simulink model "Sway_control_test"  (R2021a)
settings: Solver=VariableStepAuto  StartTime=0.0  StopTime=100.0  MaxStep=1e-3  RelTol=1e-3
values from neighbouring files (symbols this model uses):
  bEtd = (btd + btm*it^2)/rtd^2    (= 21607.2)    [Data.m]
  g = 9.80665    [Data.m]
  it = 30    [Data.m]
  MEtd = (Jtd + Jtm_tb*it^2)/rtd^2    (= 30000)    [Data.m]
  Ms = 15000    [Data.m]
  rtd = 0.5    [Data.m]
settings Model: Creator=ThnkPad  LastModifiedBy=ThnkPad

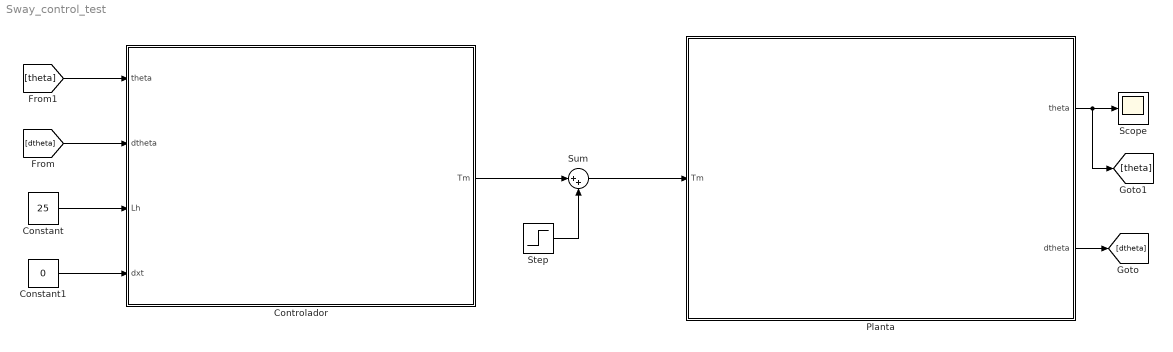
== system Sway_control_test ==
  Constant : Constant  Value=25
  Constant1 : Constant  Value=0
  Controlador : Subsystem
  Planta : Subsystem
  Scope : Scope
  Step : Step  Before=100  After=0  SampleTime=0
  Sum : Sum  Inputs=|++
  wires:
  Planta/1(theta) -> [theta], Scope/1
  Sum/1 -> Planta/1(Tm)
  Controlador/1(Tm) -> Sum/1
  Step/1 -> Sum/2
  Constant/1 -> Controlador/3(Lh)
  Planta/2(dtheta) -> [dtheta]
  [dtheta] -> Controlador/2(dtheta)
  [theta] -> Controlador/1(theta)
  Constant1/1 -> Controlador/4(dxt)

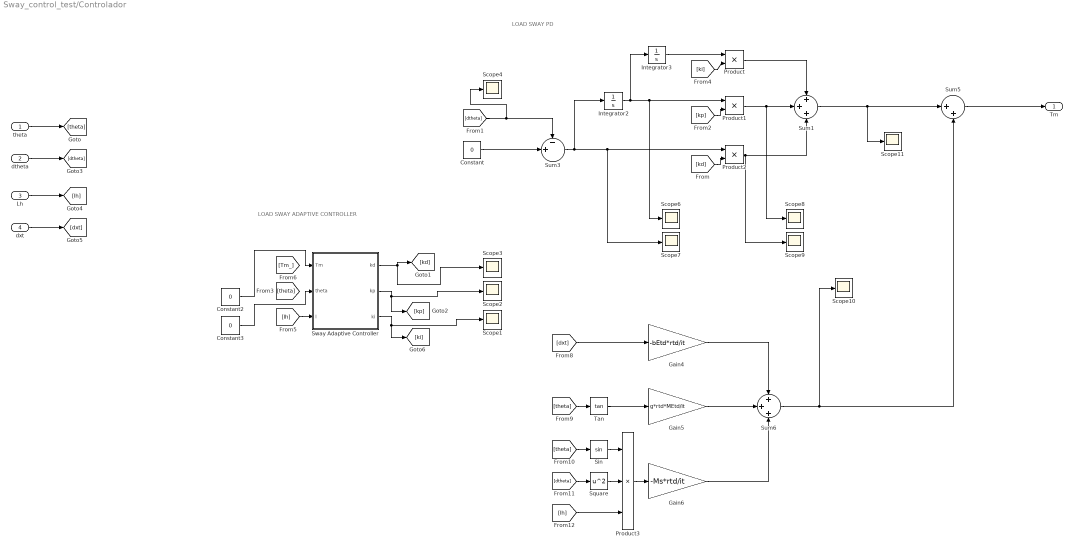
== system Sway_control_test/Controlador ==
  note: LOAD SWAY ADAPTIVE CONTROLLER
  note: LOAD SWAY PD
  theta : Inport
  dtheta : Inport  Port=2
  Lh : Inport  Port=3
  dxt : Inport  Port=4
  Constant : Constant  Value=0
  Constant2 : Constant  Value=0
  Constant3 : Constant  Value=0
  Gain4 : Gain  Gain=-bEtd*rtd/it
  Gain5 : Gain  Gain=g*rtd*MEtd/it
  Gain6 : Gain  Gain=-Ms*rtd/it
  Integrator2 : Integrator
  Integrator3 : Integrator
  Product : Product
  Product1 : Product
  Product2 : Product
  Product3 : Product  Inputs=3
  Scope{1..4,6..11} (10 alike) : Scope
  Sin : Trigonometry
  Square : Math  Operator=square  SaturateOnIntegerOverflow=on
  Sum1 : Sum  Inputs=+++
  Sum3 : Sum  Inputs=-+|
  Sum5 : Sum  Inputs=|++
  Sum6 : Sum  Inputs=+++
  Sway Adaptive Controller : Subsystem
  Tan : Trigonometry  Operator=tan
  Tm : Outport
  wires:
  Sway Adaptive Controller/3(ki) -> Scope1/1, [ki]
  Sway Adaptive Controller/2(kp) -> [kp], Scope2/1
  Integrator2/1 -> Integrator3/1, Scope6/1, Product1/1
  [dxt] -> Gain4/1
  [theta] -> Sin/1
  Product1/1 -> Scope8/1, Sum1/2
  Sum6/1 -> Sum5/2, Scope10/1
  Integrator3/1 -> Product/1
  [kp] -> Product1/2
  [dtheta] -> Scope4/1, Sum3/1
  Sway Adaptive Controller/1(kd) -> Scope3/1, [kd]
  Sum3/1 -> Scope7/1, Product2/1, Integrator2/1
  [lh] -> Sway Adaptive Controller/3(l)
  Sin/1 -> Product3/1
  Product3/1 -> Gain6/1
  Product2/1 -> Sum1/3, Scope9/1
  Sum5/1 -> Tm/1
  Constant2/1 -> Sway Adaptive Controller/1(Tm)
  Product/1 -> Sum1/1
  Sum1/1 -> Sum5/1, Scope11/1
  [ki] -> Product/2
  Constant/1 -> Sum3/2
  Constant3/1 -> Sway Adaptive Controller/2(theta)
  [theta] -> Tan/1
  Gain4/1 -> Sum6/1
  [kd] -> Product2/2
  Square/1 -> Product3/2
  Gain5/1 -> Sum6/2
  Tan/1 -> Gain5/1
  [dtheta] -> Square/1
  [lh] -> Product3/3
  Gain6/1 -> Sum6/3
  theta/1 -> [theta]
  dtheta/1 -> [dtheta]
  Lh/1 -> [lh]
  dxt/1 -> [dxt]

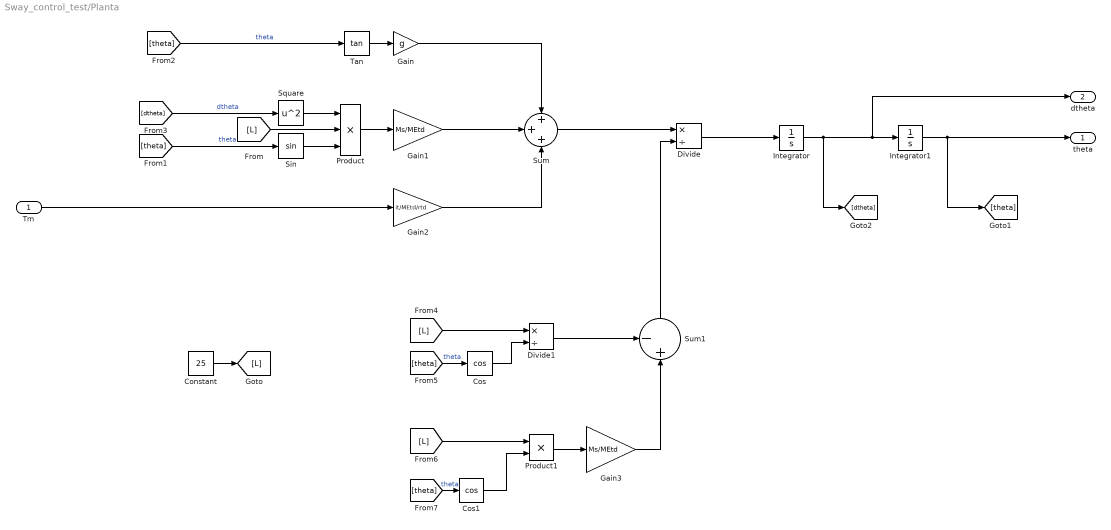
== system Sway_control_test/Planta ==
  Tm : Inport
  Constant : Constant  Value=25
  Cos : Trigonometry  Operator=cos
  Cos1 : Trigonometry  Operator=cos
  Divide : Product  Inputs=*/
  Divide1 : Product  Inputs=*/
  Gain : Gain  Gain=g
  Gain1 : Gain  Gain=Ms/MEtd
  Gain2 : Gain  Gain=it/MEtd/rtd
  Gain3 : Gain  Gain=Ms/MEtd
  Integrator : Integrator
  Integrator1 : Integrator
  Product : Product  Inputs=3
  Product1 : Product
  Sin : Trigonometry
  Square : Math  Operator=square  SaturateOnIntegerOverflow=on
  Sum : Sum  Inputs=+++
  Sum1 : Sum  Inputs=-+|
  Tan : Trigonometry  Operator=tan
  theta : Outport
  dtheta : Outport  Port=2
  wires:
  Sum1/1 -> Divide/2
  Sin/1 -> Product/3
  Integrator/1 -> [dtheta], dtheta/1, Integrator1/1
  Square/1 -> Product/1
  Gain3/1 -> Sum1/2
  [theta] -> Sin/1  "theta"
  Sum/1 -> Divide/1
  Gain/1 -> Sum/1
  Product1/1 -> Gain3/1
  Gain1/1 -> Sum/2
  Divide/1 -> Integrator/1
  [theta] -> Cos1/1  "theta"
  Constant/1 -> [L]
  Tm/1 -> Gain2/1
  Cos/1 -> Divide1/2
  [theta] -> Cos/1  "theta"
  Integrator1/1 -> theta/1, [theta]
  Tan/1 -> Gain/1
  Cos1/1 -> Product1/2
  [theta] -> Tan/1  "theta"
  Divide1/1 -> Sum1/1
  [L] -> Product/2
  Product/1 -> Gain1/1
  [dtheta] -> Square/1  "dtheta"
  Gain2/1 -> Sum/3
  [L] -> Divide1/1
  [L] -> Product1/1

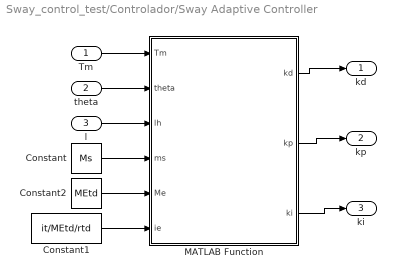
== system Sway_control_test/Controlador/Sway Adaptive Controller ==
  Tm : Inport
  theta : Inport  Port=2
  l : Inport  Port=3
  Constant : Constant  Value=Ms
  Constant1 : Constant  Value=it/MEtd/rtd
  Constant2 : Constant  Value=MEtd
  MATLAB Function : MATLAB Function  TreatAsAtomicUnit=on
  kd : Outport
  kp : Outport  Port=2
  ki : Outport  Port=3
  wires:
  Tm/1 -> MATLAB Function/1(Tm)
  theta/1 -> MATLAB Function/2(theta)
  MATLAB Function/2(kp) -> kp/1
  MATLAB Function/1(kd) -> kd/1
  l/1 -> MATLAB Function/3(lh)
  Constant/1 -> MATLAB Function/4(ms)
  MATLAB Function/3(ki) -> ki/1
  Constant1/1 -> MATLAB Function/6(ie)
  Constant2/1 -> MATLAB Function/5(Me)

== matlab function Sway_control_test/Controlador/Sway Adaptive Controller/MATLAB Function ==
  data: Tm input; kd output; theta input; kp output; lh input; ms input; Me input; ki output; ie input
function [kd, kp, ki] = get_sway_adaptive_gains(Tm,theta,lh, ms,Me, ie)

g=9.81;
A21 = -cos(theta) * g / lh + sin(theta) * Tm *ie/lh;
B2 = -cos(theta) *ie/lh;

A21_1=-(ms*lh*cos(theta)/Me-lh/cos(theta))^(-2);
A21_2=(ms*lh/Me*sin(theta)-lh*(cos(theta)^(-2)*sin(theta)))*ie*Tm;
A21=A21_1*A21_2;
B2=ie/(ms*lh*cos(theta)/Me-lh/cos(theta));


eta=2.5;
w=5;

kd=w*eta/B2;
kp=(eta*w^2+A21)/B2;
ki=w^3/B2;

kd=2*0.8*w/B2;
kp=(w^2-A21)/B2;
ki=0;

end
